simulink model "ex3"  (R2020a)
settings: Solver=VariableStepAuto  StartTime=0.0  StopTime=10.0  RelTol=1e-3
settings Model: OrderedModelArguments=off  Creator=Admin  LastModifiedBy=Admin

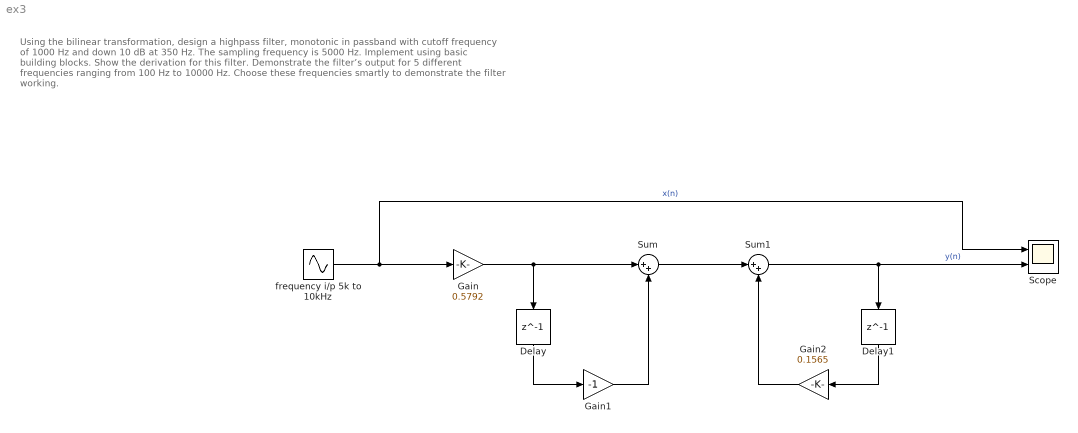
== system ex3 ==
  note: Using the bilinear transformation, design a highpass filter,
      | monotonic in passband with cutoff frequency of 1000 Hz and down 10 dB at 350 Hz.
      | The sampling frequency is 5000 Hz. Implement using basic building blocks. Show the
      | derivation for this filter. Demonstrate the filter’s output for 5 different frequencies
      | ranging from 100 Hz to 10000 Hz. Choose these frequencies smartly to demonstrate
      | the filter working.
  Delay : Delay  DelayLength=1
  Delay1 : Delay  DelayLength=1
  Gain : Gain  Gain=0.5792
  Gain1 : Gain  Gain=-1
  Gain2 : Gain  Gain=0.1565
  Scope : Scope  NumInputPorts=2
  Sum : Sum  Inputs=|++
  Sum1 : Sum  Inputs=|++
  frequency i/p 5k to 10kHz : Sin  Frequency=10000*6.28  SampleTime=2*10^-4
  wires:
  frequency i/p 5k to 10kHz/1 -> Gain/1, Scope/1  "x(n)"
  Gain/1 -> Sum/1, Delay/1
  Delay/1 -> Gain1/1
  Gain1/1 -> Sum/2
  Sum/1 -> Sum1/1
  Sum1/1 -> Delay1/1, Scope/2  "y(n)"
  Delay1/1 -> Gain2/1
  Gain2/1 -> Sum1/2
